simulink model "Question_1"  (R2024b)
settings: Solver=VariableStepAuto  StartTime=0.0  StopTime=10.0  RelTol=1e-3
model workspace (MAT data in the model file):
  Cd = 1
  Cs = 2
  M = 10
settings Model: Creator=Sagar  LastModifiedBy=Sagar

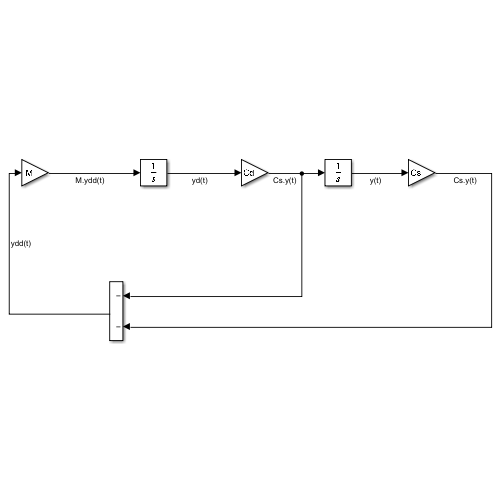
[thumbnail: Simulink's stored preview of the top-level diagram]
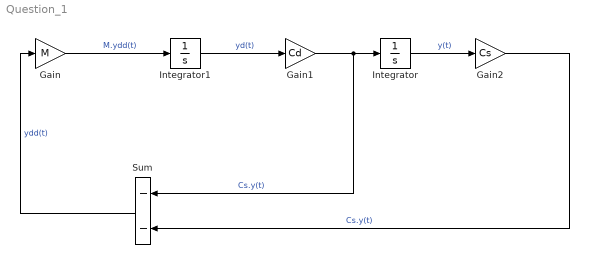
== system Question_1 ==
  Gain : Gain  Gain=M
  Gain1 : Gain  Gain=Cd
  Gain2 : Gain  Gain=Cs
  Integrator : Integrator
  Integrator1 : Integrator
  Sum : Sum  Inputs=--
  wires:
  Integrator/1 -> Gain2/1  "y(t)"
  Gain2/1 -> Sum/2  "Cs.y(t)"
  Sum/1 -> Gain/1  "ydd(t)"
  Integrator1/1 -> Gain1/1  "yd(t)"
  Gain/1 -> Integrator1/1  "M.ydd(t)"
  Gain1/1 -> Sum/1, Integrator/1  "Cs.y(t)"
